simulink model "BallAndBeam"  (R2020a)
settings: Solver=VariableStepAuto  StartTime=0.0  StopTime=100  RelTol=1e-3
libraries: ctsmodel x1
settings Model: Creator=10564  LastModifiedBy=10564

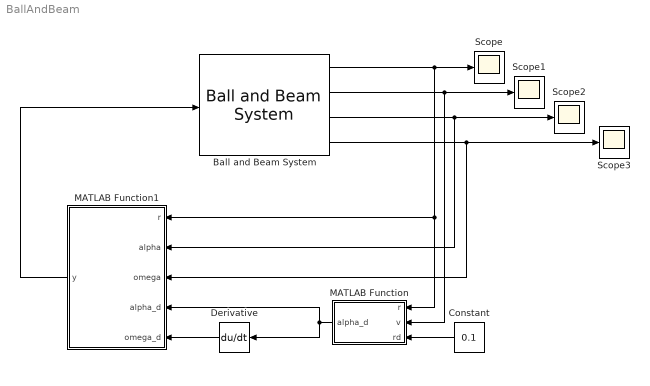
== system BallAndBeam ==
  Ball and Beam System : ctsmodel/Ball and Beam System/Ball and Beam System  Mba=0.11  R=0.015  J=0.00001  Mbe=0.4  L=0.4
      settings: SourceProductName=Control System Model Toolbox
  Constant : Constant  Value=0.1
  Derivative : Derivative
  MATLAB Function : MATLAB Function  TreatAsAtomicUnit=on
  MATLAB Function1 : MATLAB Function  TreatAsAtomicUnit=on
  Scope{,1..3} (4 alike) : Scope
  wires:
  Ball and Beam System/1 -> MATLAB Function/1(r), MATLAB Function1/1(r), Scope/1
  Ball and Beam System/2 -> MATLAB Function/2(v), Scope1/1
  Ball and Beam System/3 -> MATLAB Function1/2(alpha), Scope2/1
  Ball and Beam System/4 -> MATLAB Function1/3(omega), Scope3/1
  MATLAB Function/1(alpha_d) -> MATLAB Function1/4(alpha_d), Derivative/1
  Derivative/1 -> MATLAB Function1/5(omega_d)
  MATLAB Function1/1(y) -> Ball and Beam System/1
  Constant/1 -> MATLAB Function/3(rd)

== matlab function BallAndBeam/MATLAB Function1 ==
  data: r input; y output; alpha input; omega input; alpha_d input; omega_d input
function y = fcn(r, alpha, omega, alpha_d, omega_d)

m = 0.11;
M = 0.4;
L = 0.4;
g = 9.81;

k3=1;
k4=2;

e3 = alpha - alpha_d;
e4 = omega-omega_d + k3*e3;

y = -(k4*e4+k3*(omega-omega_d)+e3)*(m*(L-r)^2+1/3*M*L^2)+(m*g*(L-r)+0.5*M*g*L);

== matlab function BallAndBeam/MATLAB Function ==
  data: r input; alpha_d output; v input; rd input
function alpha_d = fcn(r, v, rd)

m = 0.11;
R = 0.015;
J = 0.00001;
g = 9.81;

k1=1;
k2=2;

e1 = r - rd;
e2 = v + k1*e1;

alpha_d = -(k2*e2+k1*v+e1)*(m+J/R^2)/(m*g);
